simulink model "nonlinearfunctionsimulink"  (R2022b)
settings: Solver=VariableStepAuto  StartTime=0.0  StopTime=100  RelTol=1e-3
settings Model: Creator=Windows 10  LastModifiedBy=Windows 10

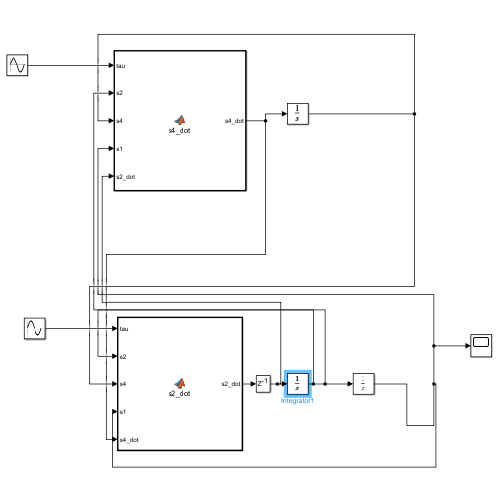
[thumbnail: Simulink's stored preview of the top-level diagram]
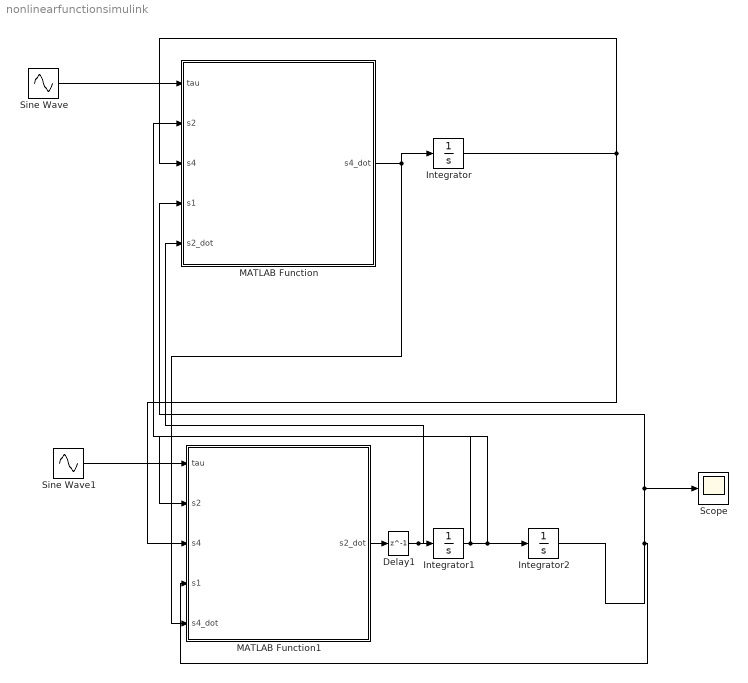
== system nonlinearfunctionsimulink ==
  Delay1 : Delay  DelayLength=1  InitialCondition=0
  Integrator : Integrator
  Integrator1 : Integrator
  Integrator2 : Integrator
  MATLAB Function : MATLAB Function  TreatAsAtomicUnit=on
  MATLAB Function1 : MATLAB Function  TreatAsAtomicUnit=on
  Scope : Scope
  Sine Wave : Sin  Phase=pi/4  SampleTime=0
  Sine Wave1 : Sin  Phase=pi/4  SampleTime=0
  wires:
  MATLAB Function/1(s4_dot) -> Integrator/1, MATLAB Function1/5(s4_dot)
  Integrator/1 -> MATLAB Function/3(s4), MATLAB Function1/3(s4)
  MATLAB Function1/1(s2_dot) -> Delay1/1
  Integrator1/1 -> MATLAB Function/2(s2), Integrator2/1, MATLAB Function1/2(s2)
  Sine Wave/1 -> MATLAB Function/1(tau)
  Sine Wave1/1 -> MATLAB Function1/1(tau)
  Integrator2/1 -> Scope/1, MATLAB Function/4(s1), MATLAB Function1/4(s1)
  Delay1/1 -> MATLAB Function/5(s2_dot), Integrator1/1

== matlab function nonlinearfunctionsimulink/MATLAB Function1 ==
  data: tau input; s2_dot output; s2 input; s4 input; s1 input; s4_dot input
function s2_dot = s2_dot(tau,s2,s4,s1,s4_dot)
b=0.01;
m=5;
l_g=0.4;
g=10;
r=0.2;
I_p=0.2;
s2_dot=(-tau-(b*(s2-s4))+(m*l_g*g*sin(s1))-(m*r*l_g*cos(s1)*s4_dot))/((m*(l_g-g^2))+I_p);

== matlab function nonlinearfunctionsimulink/MATLAB Function ==
  data: tau input; s4_dot output; s2 input; s4 input; s1 input; s2_dot input
function s4_dot = s4_dot(tau,s2,s4,s1,s2_dot)
b=0.01;
m=5;
r=0.2;
l_g=0.4;
M=10;
I_p=0.2;
s4_dot=(tau+(b*(s2-s4))+m*r*l_g*sin(s1)*(s2^2)-(m*r*l_g*cos(s1)*s2_dot))/(((m+M)*(r^2))+I_p);
